simulink model "PID"  (R2025b)
settings: Solver=VariableStepAuto  StartTime=0.0  StopTime=10  RelTol=1e-3
settings Model: Creator=Entrar  LastModifiedBy=Usuario

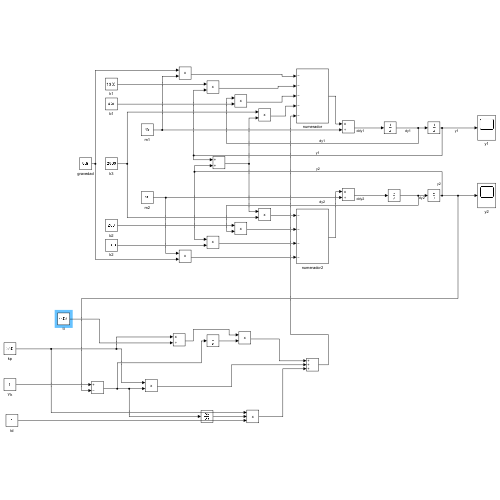
[thumbnail: Simulink's stored preview of the top-level diagram]
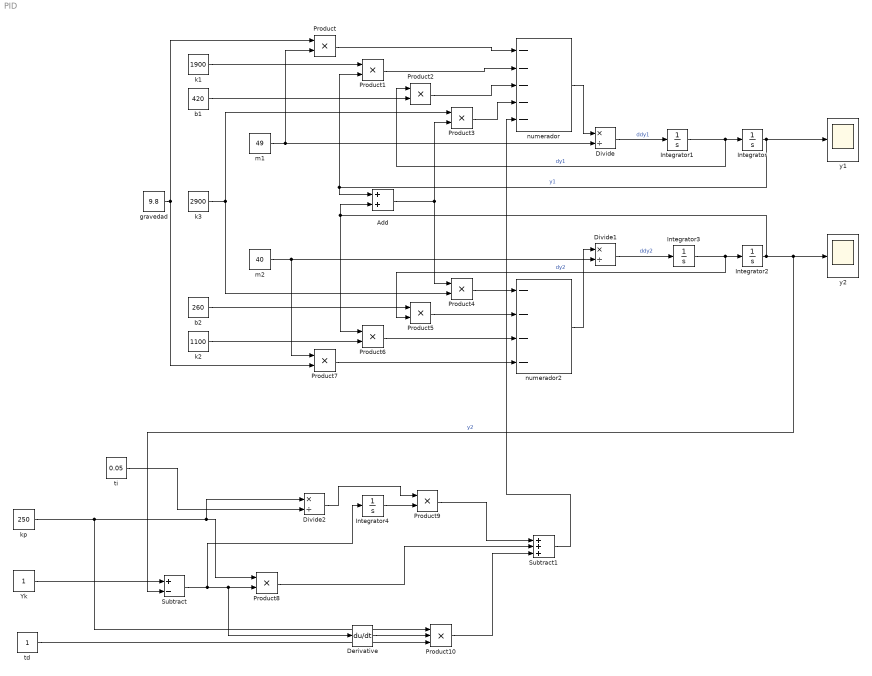
== system PID ==
  Add : Sum
  Derivative : Derivative
  Divide : Product  Inputs=*/
  Divide1 : Product  Inputs=*/
  Divide2 : Product  Inputs=*/
  Integrator{,1..4} (5 alike) : Integrator
  Product{,1..9} (10 alike) : Product
  Product10 : Product  Inputs=3
  Subtract : Sum  Inputs=+-
  Subtract1 : Sum  Inputs=+++
  Yk : Constant
  b1 : Constant  Value=420
  b2 : Constant  Value=260
  gravedad : Constant  Value=9.8
  k1 : Constant  Value=1900
  k2 : Constant  Value=1100
  k3 : Constant  Value=2900
  kp : Constant  Value=250
  m1 : Constant  Value=49
  m2 : Constant  Value=40
  numerador : Sum  Inputs=-----
  numerador2 : Sum  Inputs=----
  td : Constant
  ti : Constant  Value=0.05
  y1 : Scope
      settings: Description=y  ActiveDisplayYMinimum=-1.4767335604821041  ActiveDisplayYMaximum=0.093021611701813445
  y2 : Scope
      settings: Description=y  ActiveDisplayYMinimum=-0.18602344395032186  ActiveDisplayYMaximum=1.1370692900759372
  wires:
  Integrator1/1 -> Product2/1, Integrator/1  "dy1"
  gravedad/1 -> Product/1, Product7/2
  m1/1 -> Product/2, Divide/2
  Product/1 -> numerador/1
  Integrator/1 -> y1/1, Add/1, Product1/2  "y1"
  Divide/1 -> Integrator1/1  "ddy1"
  numerador/1 -> Divide/1
  k1/1 -> Product1/1
  Product1/1 -> numerador/2
  b1/1 -> Product2/2
  Product2/1 -> numerador/3
  Integrator3/1 -> Product5/2, Integrator2/1  "dy2"
  Integrator2/1 -> Product6/1, Add/2, Subtract/2, y2/1  "y2"
  Add/1 -> Product4/1, Product3/2
  k3/1 -> Product3/1, Product4/2
  Product3/1 -> numerador/4
  Divide1/1 -> Integrator3/1  "ddy2"
  numerador2/1 -> Divide1/1
  Product4/1 -> numerador2/1
  b2/1 -> Product5/1
  Product5/1 -> numerador2/2
  k2/1 -> Product6/2
  Product6/1 -> numerador2/3
  m2/1 -> Product7/1, Divide1/2
  Product7/1 -> numerador2/4
  Yk/1 -> Subtract/1
  Subtract/1 -> Integrator4/1, Derivative/1, Product8/2
  Subtract1/1 -> numerador/5
  kp/1 -> Product10/1, Divide2/1, Product8/1
  Product8/1 -> Subtract1/2
  Product9/1 -> Subtract1/1
  Integrator4/1 -> Product9/2
  ti/1 -> Divide2/2
  Divide2/1 -> Product9/1
  td/1 -> Product10/3
  Derivative/1 -> Product10/2
  Product10/1 -> Subtract1/3
